simulink model "HalfScaraSinusoidalMotion"  (Simulink 6.5)
settings: Solver=ode3  StartTime=0.0  StopTime=inf  FixedStep=0.05  RelTol=1e-3
libraries: RT x1, vrlib x1
settings Model: Creator=Tim Salcudean  LastModifiedBy=Tim Salcudean
settings SolverCC: ZeroCrossControl=DisableAll
settings DebuggingCC: MaxConsecutiveZCsMsg=warning  SolverPrmCheckMsg=none  MultiTaskDSMMsg=warning  MultiTaskCondExecSysMsg=none  StrictBusMsg=None
settings RTWCC: IncludeERTFirstTime=on

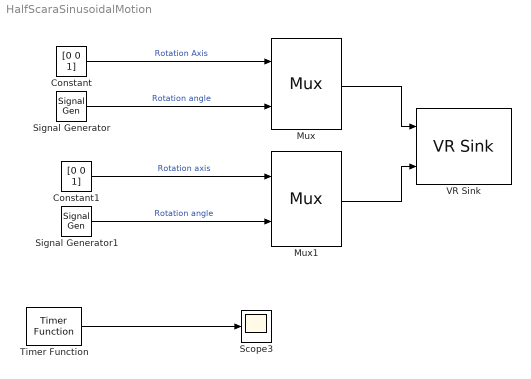
== system HalfScaraSinusoidalMotion ==
  Constant : Constant  Value=[0 0 1]  OutDataType=sfix(16)  ConRadixGroup=Use specified scaling  OutScaling=2^0  SampleTime=inf  FramePeriod=inf
  Constant1 : Constant  Value=[0 0 1]  OutDataType=sfix(16)  ConRadixGroup=Use specified scaling  OutScaling=2^0  SampleTime=inf  FramePeriod=inf
  Mux : Mux  Inputs=2
      settings: DisplayOption=signals
  Mux1 : Mux  Inputs=2
      settings: DisplayOption=signals
  Scope3 : Scope
      settings: YMin=87252  YMax=87262  SaveName=ScopeData2
  Signal Generator : SignalGenerator  Amplitude=3.141/2  Frequency=0.2
  Signal Generator1 : SignalGenerator  Amplitude=3.141/2  Frequency=0.2
  Timer Function : RT/Timer Function  Priority=283954632  step=50  priority=HIGH  ThPriority=TIME CRITICAL
  VR Sink : vrlib/VR Sink  SampleTime=-1  ViewEnable=on  RemoteChange=off  RemoteView=off  FieldsWritten=Link1.rotation.4.1.double#Link2.rotation.4.1.double  WorldFileName=HalfScara.WRL  AutoView=off  FigureProperties={}
  wires:
  Timer Function/1 -> Scope3/1
  Constant/1 -> Mux/1  "Rotation Axis"
  Signal Generator/1 -> Mux/2  "Rotation angle"
  Constant1/1 -> Mux1/1  "Rotation axis"
  Signal Generator1/1 -> Mux1/2  "Rotation angle"
  Mux/1 -> VR Sink/1
  Mux1/1 -> VR Sink/2
